simulink model "monoaxial_model_2"  (R2023b)
settings: Solver=VariableStepAuto  StartTime=0.0  StopTime=10  RelTol=1e-3
values from neighbouring files (symbols this model uses):
  A = [0     1 ... (first row only)    [main.m]    (also in monoaxial_model.m = [Ts 0;Ts, Ts])
  B = [0; 1/Ixx]    [main.m]    (also in monoaxial_model.m = [1;0])
  C = [1 0]    [main.m]    (also in monoaxial_model.m = [1,0])
  D = 0    [monoaxial_model.m]
undefined symbols (not defined in the file or in its folder): Discrete, Time
libraries: simulink x1, ctrlSharedLib x1, slpidlib x1
settings Model: Creator=alexz  LastModifiedBy=alexz

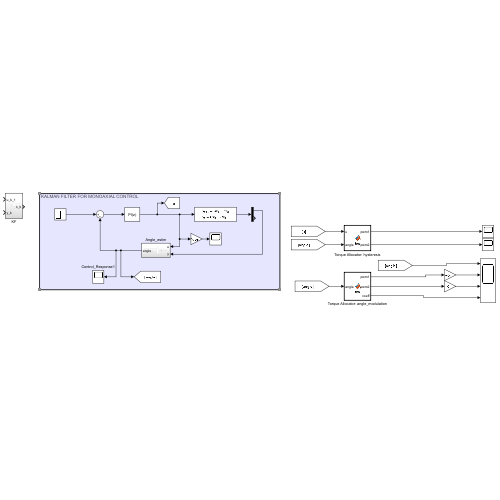
[thumbnail: Simulink's stored preview of the top-level diagram]
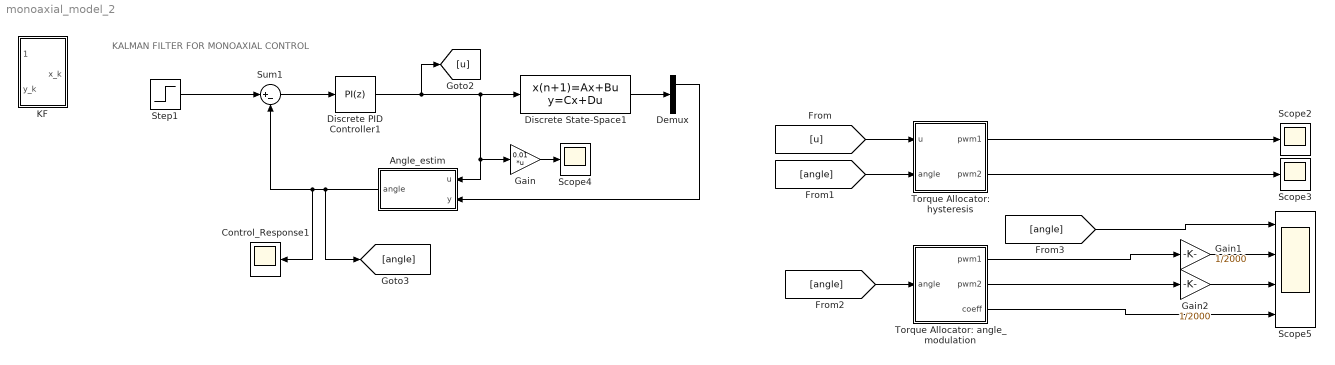
== system monoaxial_model_2 ==
  note: KALMAN FILTER FOR MONOAXIAL CONTROL
  Angle_estim : Subsystem
  Control_Response1 : Scope
  Demux : Demux  Outputs=2
  Discrete PID Controller1 : slpidlib/PID Controller  Controller=PI  Form=Parallel  TimeDomain=Discrete-time  UseExternalTs=off  SampleTime=-1  IntegratorMethod=Forward Euler  FilterMethod=Forward Euler  ControllerParametersSource=internal  P=14.0440610723537  I=209.051013385286  UseKiTs=off  D=0  N=100  UseFilter=on  TunerSelectOption=Transfer Function Based (PID Tuner App)  InitialConditionSource=internal  InitialConditionForIntegrator=0  InitialConditionForFilter=0  DifferentiatorICPrevScaledInput=0  ExternalReset=none  TrackingMode=off  Kt=1  LimitOutput=off  SatLimitsSource=internal  UpperSaturationLimit=inf  LowerSaturationLimit=-inf  LinearizeAsGain=off  AntiWindupMode=none  Kb=1  LimitIntegrator=off  UpperIntegratorSaturationLimit=inf  LowerIntegratorSaturationLimit=-inf  POutMin=[]  POutMax=[]  IOutMin=[]  IOutMax=[]  DOutMin=[]  DOutMax=[]  NOutMin=[]  NOutMax=[]  SumOutMin=[]  SumOutMax=[]  SaturationOutMin=[]  SaturationOutMax=[]  PParamMin=[]  PParamMax=[]  IParamMin=[]  IParamMax=[]  DParamMin=[]  DParamMax=[]  NParamMin=[]  NParamMax=[]  KbParamMin=[]  KbParamMax=[]  KtParamMin=[]  KtParamMax=[]  KbOutMin=[]  KbOutMax=[]  KtOutMin=[]  KtOutMax=[]  IntegratorOutMin=[]  IntegratorOutMax=[]  FilterOutMin=[]  FilterOutMax=[]  SumI1OutMin=[]  SumI1OutMax=[]  SumI2OutMin=[]  SumI2OutMax=[]  SumI3OutMin=[]  SumI3OutMax=[]  SumI4OutMin=[]  SumI4OutMax=[]  SumDOutMin=[]  SumDOutMax=[]  DifferentiatorOutMin=[]  DifferentiatorOutMax=[]  FilterDiffOutCoefMin=[]  FilterDiffOutCoefMax=[]  ReciprocalOutMin=[]  ReciprocalOutMax=[]  SumDenOutMin=[]  SumDenOutMax=[]  SumNumOutMin=[]  SumNumOutMax=[]  DivideOutMin=[]  DivideOutMax=[]  UdiffTsProdOutMin=[]  UdiffTsProdOutMax=[]  NTsProdOutMin=[]  NTsProdOutMax=[]  UintegralTsProdOutMin=[]  UintegralTsProdOutMax=[]  UngainTsProdOutMin=[]  UngainTsProdOutMax=[]  ClampingZeroOutDataTypeStr=Inherit: Inherit via back propagation  ClampingZeroOutMin=[]  ClampingZeroOutMax=[]  FilterDenConstantOutDataTypeStr=Inherit: Inherit via back propagation  FilterDenConstantOutMin=[]  FilterDenConstantOutMax=[]  PCopyOutDataTypeStr=Inherit: Inherit via back propagation  PCopyOutMin=[]  PCopyOutMax=[]  NCopyOutDataTypeStr=Inherit: Inherit via back propagation  NCopyOutMin=[]  NCopyOutMax=[]  IntegratorContinuousStateAttributes=''  IntegratorStateMustResolveToSignalObject=off  IntegratorRTWStateStorageClass=Auto  FilterContinuousStateAttributes=''  FilterStateMustResolveToSignalObject=off  FilterRTWStateStorageClass=Auto  ParallelPVariant=InternalParameters  IdealPVariant=Disabled  IVariant=InternalParameters  DVariant=Disabled  IntegratorVariant=Discrete  SatVariant=Disabled  AWVariant=Passthrough  PCopyVariant=Disabled  TRVariant=Disabled  FdbkBlocksVariant=Forward  IdealPFdbkVariant=Disabled  SatFdbkVariant=Disabled  DerivativeFilterVariant=Disabled  NVariant=Disabled  NCopyVariant=Disabled_SignalSpec  FilterICVariant=Disabled  IntegratorICVariant=InternalICs  ExternalResetVariant=Disabled  TRSumVariant=Passthrough  SumFdbkVariant=Disabled  SumVariant=Sum_PI  TsampFilterVariant=InternalTs  TsampNgainVariant=Passthrough  TsampIntegralVariant=Disabled_SignalSpec  ExternalSaturationOutDataTypeStr=Inherit: Same as second input
      settings: LibrarySourceBlock=simulink/Discrete/Discrete PID Controller
  Discrete State-Space1 : DiscreteStateSpace  A=A  B=B  C=eye(2)  D=zeros(2,1)  SampleTime=-1
  Gain : Gain  Gain=0.01  Multiplication=Matrix(K*u) (u vector)
  Gain1 : Gain  Gain=1/2000
  Gain2 : Gain  Gain=1/2000
  KF : Subsystem
  Scope2 : Scope
  Scope3 : Scope
  Scope4 : Scope
  Scope5 : Scope  NumInputPorts=4
  Step1 : Step  Time=2  Before=-1  After=0  SampleTime=0
  Sum1 : Sum  Inputs=|+-
  Torque Allocator: angle_modulation : MATLAB Function  TreatAsAtomicUnit=on
  Torque Allocator: hysteresis : MATLAB Function  TreatAsAtomicUnit=on
  wires:
  Sum1/1 -> Discrete PID Controller1/1
  Step1/1 -> Sum1/1
  Discrete State-Space1/1 -> Demux/1
  Demux/1 -> Angle_estim/2(y)
  Angle_estim/1(angle) -> [angle], Sum1/2, Control_Response1/1
  [u] -> Torque Allocator: hysteresis/1(u)
  [angle] -> Torque Allocator: hysteresis/2(angle)
  Torque Allocator: hysteresis/1(pwm1) -> Scope2/1
  Torque Allocator: hysteresis/2(pwm2) -> Scope3/1
  Discrete PID Controller1/1 -> Discrete State-Space1/1, Gain/1, Angle_estim/1(u), [u]
  Gain/1 -> Scope4/1
  [angle] -> Torque Allocator: angle_modulation/1(angle)
  [angle] -> Scope5/1
  Torque Allocator: angle_modulation/3(coeff) -> Scope5/4
  Torque Allocator: angle_modulation/1(pwm1) -> Gain1/1
  Torque Allocator: angle_modulation/2(pwm2) -> Gain2/1
  Gain1/1 -> Scope5/2
  Gain2/1 -> Scope5/3

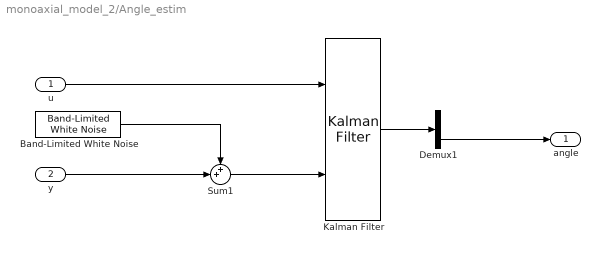
== system monoaxial_model_2/Angle_estim ==
  u : Inport
  y : Inport  Port=2
  Band-Limited White Noise : simulink/Sources/Band-Limited White Noise  Cov=[0.1]  Ts=0.1  seed=[23341]
  Demux1 : Demux  Outputs=2
  Kalman Filter : ctrlSharedLib/Kalman Filter  TimeDomain=Discrete-Time  UseCurrentEstimator=on  ModelSource=Individual A, B, C, D matrices  ModelSourceVariable=sys  A=A  B=B  C=C  D=D  NumberOfStates=2  NumberOfInputs=2  NumberOfOutputs=2  InitialEstimateSource=Dialog  X0=0  P0=10  UseK=off  UseGH=off  NumberOfProcessNoiseInputs=2  G=1  TimeInvariantG=on  H=0  TimeInvariantH=on  Q=10  TimeInvariantQ=on  R=0.01  TimeInvariantR=on  N=0  TimeInvariantN=on  AddInputPort=on  AddEnablePort=off  OutputEstimatedY=off  OutputP=off  Ts=-1
      settings: LibrarySourceBlock=slident/Estimators/Kalman Filter
  Sum1 : Sum  Inputs=++|
  angle : Outport
  wires:
  y/1 -> Sum1/2
  Demux1/2 -> angle/1
  Band-Limited White Noise/1 -> Sum1/1
  Kalman Filter/1 -> Demux1/1
  u/1 -> Kalman Filter/1
  Sum1/1 -> Kalman Filter/2

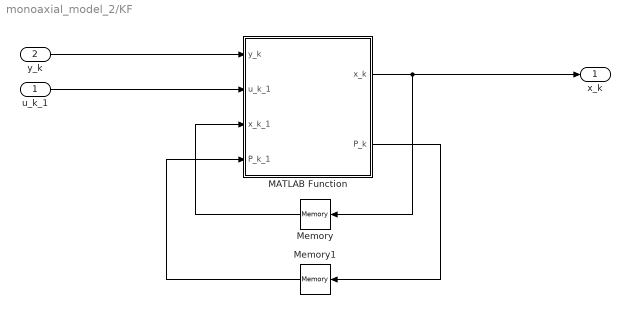
== system monoaxial_model_2/KF ==
  u_k_1 : Inport
  y_k : Inport  Port=2
  MATLAB Function : MATLAB Function  TreatAsAtomicUnit=on
  Memory : Memory
  Memory1 : Memory
  x_k : Outport
  wires:
  u_k_1/1 -> MATLAB Function/2(u_k_1)
  MATLAB Function/2(P_k) -> Memory1/1
  MATLAB Function/1(x_k) -> Memory/1, x_k/1
  y_k/1 -> MATLAB Function/1(y_k)
  Memory/1 -> MATLAB Function/3(x_k_1)
  Memory1/1 -> MATLAB Function/4(P_k_1)

== matlab function monoaxial_model_2/Torque Allocator: hysteresis ==
  data: u input; pwm1 output; pwm2 output; angle input
function [pwm1, pwm2] = fcn(u, angle)
J = 0.01;
k = 0.002;
torque = u*J;
if angle<=0
    u2 = 0;
    u1 = torque;
else 
    u2 = torque;
    u1 = 0;
end

pwm1 = min(2000, max(1000,u1/k+1500));
pwm2 = min(2000, max(1000,u2/k+1500));

== matlab function monoaxial_model_2/KF/MATLAB Function ==
  data: y_k input; u_k_1 input; x_k output; x_k_1 input; P_k_1 input; P_k output
function [x_k, P_k]  = fcn(y_k, u_k_1, x_k_1, P_k_1)
%% PARAMETERS
Ts = 0.01;
R = 100;
Q = 0.01;
A = [Ts 0;Ts, Ts];
B = [1;0];
C = [1,0];

P_k = A*P_k_1*A'+Q;
L_k = P_k*C'*(C*P_k*C'+R)^(-1);

x_k = A*x_k_1+B*u_k_1+L_k*(y_k-C*(A*x_k_1+B*u_k_1));

== matlab function monoaxial_model_2/Torque Allocator: angle_modulation ==
  data: pwm1 output; pwm2 output; angle input; coeff output
function [pwm1, pwm2, coeff] = fcn(angle)

max_angle = pi/2;
coeff = 0.5 + (angle/max_angle)/2;

 pwm1 = 1000*(1-coeff)+1000;
 pwm2 = 1000*coeff     +1000;
